simulink model "tqdtqr_rebuild_V3"  (R2021b)
settings: Solver=VariableStepAuto  StartTime=0.0  StopTime=10.0  RelTol=1e-3
undefined symbols (not defined in the file): ATQD_AfterTqMinGain_X_Deg, ATQD_APSCreepBaseTqD_X_kph, ATQD_APSCreepBaseTqD_Y_Deg, ATQD_APSCreepBaseTqR_X_kph, ATQD_APSCreepBaseTqR_Y_Deg, ATQD_APSCreepIterm_X_kph, ATQD_APSCreepIterm_Y_kph, ATQD_APSCreepPterm_X_kph, ATQD_APSCreepPterm_Y_kph, ATQD_APSDecReq_X_kph, ATQD_APSDecReq_Y_mps2, ATQD_APSDecReqCMD_X_kph, ATQD_APSDecReqTs_X_pct, ATQD_APSDecTimeGain_X_Deg, ATQD_APSDecTimeGain_Y_s, ATQD_APSReqLowSpd_X_Deg, ATQD_AutoHoldReleaseBPS_X_Deg, ATQD_AWDLoadTrqnsGain_X_kg, ATQD_AWDLoadTrqnsGain_Y_pct, ATQD_BOSEnBPSPosn_X_kph, ATQD_BOSMap_X_rpm, ATQD_BOSMap_Y_pct, ATQD_CreepBaseTqD_X_kph, ATQD_CreepBaseTqD_Y_Deg, ATQD_CreepBaseTqR_X_kph, ATQD_CreepBaseTqR_Y_Deg, ATQD_CreepBPSDisPosn_X_Deg, ATQD_CreepBPSDisPosnR_X_Deg, ATQD_CreepBPSEnPosn_X_Deg, ATQD_CreepBPSEnPosnR_X_Deg, ATQD_CreepDeltaTq_X_kph, ATQD_CreepIterm_X_kph, ATQD_CreepIterm_Y_kph, ATQD_CreepItermMaxLimit_X_pct, ATQD_CreepPreloadTime_X_kph, ATQD_CreepPreloadTq_X_kph, ATQD_CreepPreloadTq_Y_s, ATQD_CreepProtTq_X_Deg, ATQD_CreepPterm_X_kph, ATQD_CreepPterm_Y_kph, ATQD_CreepRrTqSpRat_X_rpm, ATQD_CreepRrTqSpRat_Y_Nm, ATQD_CreepTargetSpdD_X_pct, ATQD_CreepTargetSpdR_X_pct, ATQD_CreepUpLimitTq_X_rpm, ATQD_DecIneOPDHoldEnDelay_X_Deg, ATQD_DecIneOPDHoldEnDelay_Y_bar, ATQD_ECOTqMapD_X_rpm, ATQD_ECOTqMapD_Y_pct, ATQD_EMTqMapD_X_rpm, ATQD_EMTqMapD_Y_pct, ATQD_EOPDTqMapDCon_X_rpm, ATQD_EOPDTqMapDCon_Y_Deg, ATQD_EstInitVehWeight_X_c, ATQD_FAfterTqCMDGain_X_rpm, ATQD_FAfterTqCMDGain_Y_pct, ATQD_ForceLowSpd_X_Deg, ATQD_ForcePLimitSpd_X_Deg, ATQD_FrLossMAPLowV_X_rpm, ATQD_FrLossMAPLowV_Y_Nm ... (+949)
libraries: simulink x235, hcu_lib x208, tqr x63, tqd x6
(part 23 of 37)

== system tqdtqr_rebuild_V3/Input_Convert/Signal function/SWC1 SWC2 status/SWC2_Subsystem ==
  note: Fail safe switch
  note: Speed Control Mode
  note: Speed Setting Mode
  VINP_SWC2LScrollUpSta_flg : Inport
  VINP_SWC2LScrollDownSta_flg : Inport  Port=2
  VINP_SWC2LScrollPressSta_flg : Inport  Port=3
  VINP_SWC2LADASSta_flg : Inport  Port=4
  VTQD_GearActualPosn_enum : Inport  Port=5
  VVMC_ADASActive_flg : Inport  Port=6
  VVMC_LVDAACCStaInfor_flg : Inport  Port=7
  VVMC_MSAActive_flg : Inport  Port=8
  VINP_ADASACCSta_enum : Inport  Port=9
  VVMC_MeterIndSpeed_raw32 : Inport  Port=10
  VINP_ADASSLIFSpdLim_enum : Inport  Port=11
  task_time_s : Inport  Port=12
  VINP_IVIISAOffsetSpd_enum : Inport  Port=13
  VPMM_PowerSta_enum : Inport  Port=14
  VTQD_ShiftGearPosn_enum : Inport  Port=15
  VVMC_MSACtrlSta_enum : Inport  Port=16
  VINP_Distanceunit_flg : Inport  Port=17
  VINP_IVIACCAdaptiveSta_flg : Inport  Port=18
  VVMC_CCCtrlSta_enum : Inport  Port=19
  VINP_SmartEcoModeSW_flg : Inport  Port=20
  VTQD_LowIdleAccPedal_flg : Inport  Port=21
  Enable : EnablePort
  AND1 : Logic  AllPortsSameDT=off  OutDataTypeStr=boolean
  AND{8,10,12..13,17..18} (6 alike) : Logic  Inputs=3  AllPortsSameDT=off  OutDataTypeStr=boolean
  AND11 : Logic  Inputs=4  AllPortsSameDT=off  OutDataTypeStr=boolean
  AND14 : Logic  Operator=OR  AllPortsSameDT=off  OutDataTypeStr=boolean
  AND16 : Logic  Operator=OR  AllPortsSameDT=off  OutDataTypeStr=boolean
  Add1 : Sum
  Constant1 : Constant  Value=ENUM_ADASACCSTA_OVERRIDE
  Constant{89,92,94..95,110..113} (8 alike) : Constant  Value=FALSE
  Constant116 : Constant  Value=ENUM_GEARACTUALPOSN_D
  Constant117 : Constant  Value=ENUM_SWCBOTTONPRESS_LONGPRESS
  Constant118 : Constant  Value=ENUM_GEARACTUALPOSN_D
  Constant119 : Constant  Value=ENUM_SPDCTRLMODE_MSA
  Constant120 : Constant  Value=ENUM_SWCBOTTONPRESS_SHORTPRESS
  Constant121 : Constant  Value=KTQD_OvrSpdSetDownOffSet_kph
  Constant122 : Constant  Value=ENUM_SWCBOTTONPRESS_LONGPRESS
  Constant123 : Constant  Value=ENUM_SWCBOTTONPRESS_SHORTPRESS
  Constant124 : Constant  Value=ENUM_ADASACCSTA_ACTIVE
  Constant125 : Constant  Value=ENUM_ADASACCSTA_ACTIVE
  Constant126 : Constant  Value=0x0  OutDataTypeStr=uint8
  Constant127 : Constant  Value=ENUM_SPDCTRLMODE_MSA
  Constant128 : Constant  Value=ENUM_SPDCTRLMODE_ACC
  Constant129 : Constant  Value=ENUM_GEARACTUALPOSN_D
  Constant130 : Constant  Value=ENUM_SPDCTRLMODE_MSA
  Constant77 : Constant  Value=KTQD_SpdCtrlMode_enum_ovrdflg
  Constant78 : Constant  Value=KTQD_SpdCtrlMode_enum_ovrdval
  Constant90 : Constant  Value=ENUM_POWERSTA_READY
  Constant91 : Constant  Value=ENUM_SPDCTRLMODE_OFF
  Data Type Conversion : DataTypeConversion  OutDataTypeStr=boolean
  Data Type Conversion4 : DataTypeConversion  OutDataTypeStr=single
  Delay{10..13} (4 alike) : Delay  DelayLength=1  InitialCondition=uint8(0)
      settings: AttributesFormatString=%<InitialCondition>
  Delay5 : Delay  DelayLength=1  InitialCondition=single(0.0)
      settings: AttributesFormatString=%<InitialCondition>
  Detect Decrease2 : simulink/Logic and Bit Operations/Detect Decrease  vinit=boolean(0)  OutDataTypeStr=boolean
  Detect Increase1 : simulink/Logic and Bit Operations/Detect Increase  vinit=boolean(0)  OutDataTypeStr=boolean
  Detect Increase2 : simulink/Logic and Bit Operations/Detect Increase  vinit=boolean(0)  OutDataTypeStr=boolean
  Equal{1,30,41..48,50,52} (12 alike) : RelationalOperator  Operator===  OutDataTypeStr=boolean  RndMeth=Simplest
  Equal{40,49,51,53} (4 alike) : RelationalOperator  Operator=~=  OutDataTypeStr=boolean  RndMeth=Simplest
  L_ScrollPress Behavior : Subsystem
  NOT{1..4} (4 alike) : Logic  Operator=NOT  AllPortsSameDT=off  OutDataTypeStr=boolean
  OR2 : Logic  Operator=OR  Inputs=4  AllPortsSameDT=off  OutDataTypeStr=boolean
  OR{3..8} (6 alike) : Logic  Operator=OR  AllPortsSameDT=off  OutDataTypeStr=boolean
  Relational Operator3 : RelationalOperator  Operator=>  OutDataTypeStr=boolean  RndMeth=Simplest
  Road Speed Limit Convert : Subsystem
  SR_Latch4 : hcu_lib/Basic_Blocks/SR_Latch
  SR_Latch9 : hcu_lib/Basic_Blocks/SR_Latch
  Speed Control Mode : Stateflow chart  TreatAsAtomicUnit=on
  Speed Setting Mode : Subsystem
  Switch{13,15..16,19,23,25..26} (7 alike) : Switch  Criteria=u2 ~= 0
      settings: AttributesFormatString=%<Criteria>
  VTQD_IVIISAOffsetSpdCHOOSE_flg : Subsystem
  VTQD_SWC2ResUpSta_flg : Outport
  VTQD_SWC2SetdownSta_flg : Outport  Port=2
  VTQD_SWC2CancelSta_flg : Outport  Port=3
  VTQD_SWC2LADASSta_flg : Outport  Port=4
  VTQD_SpdLim4SetSpd_raw32 : Outport  Port=5
  VTQD_SpdCtrlMode_enum : Outport  Port=6
  VTQD_SWC2SpdCtrlSta_flg : Outport  Port=7
  VTQD_SWC2SetSpd_kph : Outport  Port=8
  VTQD_SWC2ScrollUpSta_flg : Outport  Port=9
  wires:
  [VVMC_MSACtrlSta_enum] -> L_ScrollPress Behavior/3(VVMC_MSACtrlSta_enum)
  VTQD_LowIdleAccPedal_flg/1 -> [VTQD_LowIdleAccPedal_flg]
  AND1/1 -> AND14/2
  Equal1/1 -> AND14/1
  [VTQD_LowIdleAccPedal_flg] -> NOT3/1
  [VVMC_MSAActive_flg] -> AND1/1
  [VINP_ADASACCSta_enum] -> Equal1/1
  Constant1/1 -> Equal1/2
  NOT3/1 -> AND1/2
  Constant112/1 -> [VDDM_SWC2LScrollPressSta_flg]  "VDDM_SWC2LScrollPressSta_flg"
  Constant110/1 -> [VDDM_SWC2LScrollUpSta_flg]  "VDDM_SWC2LScrollUpSta_flg"
  Constant111/1 -> [VDDM_SWC2LScrollDownSta_flg]  "VDDM_SWC2LScrollDownSta_flg"
  Constant113/1 -> [VDDM_SWC2LADASSta_flg]  "VDDM_SWC2LADASSta_flg"
  VINP_SWC2LScrollDownSta_flg/1 -> [VINP_SWC2LScrollDownSta_flg]
  VTQD_ShiftGearPosn_enum/1 -> [VTQD_ShiftGearPosn_enum]
  VINP_SWC2LScrollPressSta_flg/1 -> [VINP_SWC2LScrollPressSta_flg]
  VINP_IVIISAOffsetSpd_enum/1 -> [VINP_IVIISAOffsetSpd_enum]
  VVMC_ADASActive_flg/1 -> [VVMC_ADASActive_flg]
  VVMC_MSAActive_flg/1 -> [VVMC_MSAActive_flg]
  VVMC_MeterIndSpeed_raw32/1 -> [VVMC_MeterIndSpeed_raw32]
  VVMC_LVDAACCStaInfor_flg/1 -> [VVMC_LVDAACCStaInfor_flg]
  VINP_SWC2LScrollUpSta_flg/1 -> [VINP_SWC2LScrollUpSta_flg]
  VINP_Distanceunit_flg/1 -> [VINP_Distanceunit_flg]
  VVMC_CCCtrlSta_enum/1 -> [VVMC_CCCtrlSta_enum]
  VINP_IVIACCAdaptiveSta_flg/1 -> [VINP_IVIACCAdaptiveSta_flg]
  VINP_SmartEcoModeSW_flg/1 -> [VINP_SmartEcoModeSW_flg]
  VPMM_PowerSta_enum/1 -> [VPMM_PowerSta_enum]
  VINP_SWC2LADASSta_flg/1 -> [VINP_SWC2LADASSta_flg]
  VVMC_MSACtrlSta_enum/1 -> [VVMC_MSACtrlSta_enum]
  task_time_s/1 -> [task_time_s]
  VINP_ADASSLIFSpdLim_enum/1 -> [VINP_ADASSLIFSpdLim_enum]
  VTQD_GearActualPosn_enum/1 -> [VTQD_GearActualPosn_enum]
  VINP_ADASACCSta_enum/1 -> [VINP_ADASACCSta_enum]
  AND16/1 -> AND17/1
  OR2/1 -> [VTQD_SWC2SetDownSta_flg]  "VTQD_SWC2SetdownSta_flg"
  [VTQD_LScrollPressShort_flg] -> Speed Setting Mode/18(VTQD_LScrollPressShort_flg)
  [VTQD_SWC2ScrollUpSta_enum] -> Delay10/1
  [VTQD_GearActualPosn_enum] -> Delay12/1
  Switch25/1 -> [VTQD_SWC2ScrollDownSta_flg]  "VTQD_SWC2ScrollDownSta_flg"
  OR3/1 -> [VTQD_SWC2ResUpSta_flg]  "VTQD_SWC2ResUpSta_flg"
  Switch26/1 -> [VTQD_SWC2LScrollPressSta_flg]  "VTQD_SWC2LScrollPressSta_flg"
  Constant91/1 -> Switch15/3
  [VINP_ADASACCSta_enum] -> Equal50/1
  Constant89/1 -> Switch23/1
  [VDDM_SWC2LScrollDownSta_flg] -> Switch25/2
  [VTQD_ShiftGearPosn_enum] -> Speed Setting Mode/2(VTQD_ShiftGearPosn_enum)
  AND17/1 -> OR2/4, [VTQD_SetRoadSpdLim_flg]  "VTQD_SetRoadSpdLim_flg"
  Constant78/1 -> Switch13/1
  [VTQD_SpdCtrlMode_enum] -> Equal43/1
  [VDDM_SWC2LScrollUpSta_flg] -> Switch23/2
  Constant128/1 -> Equal46/2
  [VTQD_SWC2ScrollUpSta_flg] -> Detect Increase1/1
  OR6/1 -> AND8/3
  Equal51/1 -> OR5/1
  Equal52/1 -> AND12/3
  Constant95/1 -> Switch16/1
  [VINP_SWC2LScrollUpSta_flg] -> Switch23/3
  [VTQD_SWC2ScrollUpSta_enum] -> Equal48/1
  [VTQD_SpdCtrlMode_enum] -> Equal52/1
  AND8/1 -> SR_Latch4/1
  [VTQD_SWC2ScrollUpSta_enum] -> Equal47/1
  Delay10/1 -> Equal41/1
  [VVMC_MSAActive_flg] -> NOT4/1
  SR_Latch9/1 -> OR5/2
  Road Speed Limit Convert/1(VTQD_RoadSpdLim_raw32) -> [VTQD_RoadSpdLim_raw32]
  Equal42/1 -> AND18/2
  [VINP_SWC2LScrollDownSta_flg] -> Switch25/3
  Constant122/1 -> Equal47/2
  Constant119/1 -> Equal44/2
  Equal41/1 -> OR8/1
  [VVMC_MSAActive_flg] -> AND12/2
  [VTQD_SWC2LScrollPressSta_flg] -> L_ScrollPress Behavior/1(VTQD_SWC2LScrollPressSta_flg)
  VTQD_IVIISAOffsetSpdCHOOSE_flg/1(VTQD_IVIISAOffsetSpdCHOOSE_flg) -> [VTQD_IVIISAOffsetSpdCHOOSE_flg]
  [VPMM_PowerSta_enum] -> Equal30/1
  L_ScrollPress Behavior/1(VTQD_LScrollPressShort_flg) -> [VTQD_LScrollPressShort_flg]  "VTQD_LScrollPressShort_flg"
  [VTQD_SpdCtrlMode_enum] -> Equal46/1
  Speed Control Mode/1(VTQD_SpdCtrlMode_enum) -> Switch13/3
  Constant77/1 -> Switch13/2
  [VINP_IVIISAOffsetSpd_enum] -> VTQD_IVIISAOffsetSpdCHOOSE_flg/1(VTQD_IVIISAOffsetSpd_enum)
  Data Type Conversion4/1 -> [VTQD_SWC2SetSpd_kph]  "VTQD_SWC2SetSpd_kph"
  Constant90/1 -> Equal30/2
  Constant94/1 -> Switch26/1
  [VTQD_Set2MeterSpd_flg] -> Speed Setting Mode/16(VTQD_Set2MeterSpd_flg)
  Equal45/1 -> OR8/2
  [VINP_ADASSLIFSpdLim_enum] -> Speed Setting Mode/7(VINP_ADASSLIFSpdLim_enum)
  [VINP_SWC2LScrollPressSta_flg] -> Switch26/3
  Equal44/1 -> AND18/3
  Equal30/1 -> Switch15/2
  [VINP_SWC2LADASSta_flg] -> Switch16/3
  [VDDM_SWC2LScrollPressSta_flg] -> Switch26/2
  AND14/1 -> AND13/2
  AND13/1 -> [VTQD_Set2MeterSpd_flg], OR2/3  "VTQD_Set2MeterSpd_flg"
  [VTQD_GearActualPosn_enum] -> Equal42/1
  Equal40/1 -> AND18/1
  Add1/1 -> Relational Operator3/2
  Constant116/1 -> Equal40/2
  Detect Decrease2/1 -> SR_Latch4/2
  Equal46/1 -> AND10/3
  [VVMC_ADASActive_flg] -> AND8/1
  Delay5/1 -> Add1/2
  [VINP_ADASACCSta_enum] -> Delay13/1
  [VTQD_SWC2CANCELSta_flg] -> NOT1/1
  Constant127/1 -> Equal43/2
  OR8/1 -> Detect Decrease2/1
  [VTQD_SWC2ScrollUpSta_enum] -> Delay11/1
  Constant124/1 -> Equal49/2
  Constant117/1 -> Equal41/2
  L_ScrollPress Behavior/2("VTQD_LScrollPressLong_flg\t") -> [VTQD_LScrollPressLong_flg]  "VTQD_LScrollPressLong_flg"
  [VVMC_MeterIndSpeed_raw32] -> Relational Operator3/1
  Constant123/1 -> Equal48/2
  Constant125/1 -> Equal50/2
  Constant120/1 -> Equal45/2
  [VTQD_LScrollPressLong_flg] -> AND11/2
  [VTQD_SWC2SetSpd_kph] -> Delay5/1
  Equal53/1 -> AND17/3
  Constant126/1 -> Equal53/2
  Equal47/1 -> OR4/1
  OR5/1 -> [VTQD_SWC2CANCELSta_flg]  "VTQD_SWC2CancelSta_flg"
  [VVMC_MSAActive_flg] -> AND16/2
  [VTQD_GearActualPosn_enum] -> Equal51/1
  AND12/1 -> SR_Latch9/1
  Constant92/1 -> Switch25/1
  Speed Setting Mode/2(VTQD_SWC2ScrollUpSta_enum) -> [VTQD_SWC2ScrollUpSta_enum]
  Equal49/1 -> AND10/1
  [VVMC_ADASActive_flg] -> AND16/1
  [VTQD_LScrollPressLong_flg] -> AND12/1
  Constant121/1 -> Add1/1
  [VPMM_PowerSta_enum] -> Speed Control Mode/1(VPMM_PowerSta_enum)
  Constant129/1 -> Equal51/2
  [VTQD_SpdLim4SetSpd_raw32] -> Speed Setting Mode/12(VTQD_SpdLim4SetSpd_raw32)
  NOT1/1 -> AND11/1
  AND10/1 -> OR2/2
  [VINP_ADASSLIFSpdLim_enum] -> Road Speed Limit Convert/1(VINP_ADASSLIFSpdLim_enum)
  [VTQD_SWC2LADASSta_flg] -> Speed Control Mode/4(VTQD_SWC2LADASSta_flg)
  [VINP_Distanceunit_flg] -> Road Speed Limit Convert/4(VINP_Distanceunit_flg)
  Delay12/1 -> Equal40/1
  NOT4/1 -> AND11/4
  [VTQD_ShiftGearPosn_enum] -> Road Speed Limit Convert/5(VTQD_ShiftGearPosn_enum)
  [VVMC_MSACtrlSta_enum] -> Speed Control Mode/5(VVMC_MSACtrlSta_enum)
  Relational Operator3/1 -> AND13/1
  [VTQD_ShiftGearPosn_enum] -> Speed Control Mode/3(VTQD_ShiftGearPosn_enum)
  [VVMC_CCCtrlSta_enum] -> Speed Setting Mode/5(VVMC_CCCtrlSta_enum)
  Equal50/1 -> AND10/2
  [VTQD_SetRoadSpdLim_flg] -> OR7/2
  [VTQD_SpdCtrlMode_enum] -> Equal44/1
  [VVMC_MSACtrlSta_enum] -> Speed Setting Mode/6(VVMC_MSACtrlSta_enum)
  [VTQD_SpdCtrlMode_enum] -> Speed Setting Mode/3(VTQD_SpdCtrlMode_enum)
  [VTQD_SetRoadSpdLim_flg] -> Speed Setting Mode/17(VTQD_SetRoadSpdLim_flg)
  Equal43/1 -> AND11/3
  [task_time_s] -> L_ScrollPress Behavior/2(TASK_TIME)
  Detect Increase1/1 -> OR6/1
  OR7/1 -> Switch19/2
  OR4/1 -> AND13/3
  [VTQD_SWC2ScrollUpSta_flg] -> Speed Setting Mode/8(VTQD_SWC2ScrollUpSta_flg)
  [task_time_s] -> Speed Setting Mode/10(task_time_s)
  Switch15/1 -> [VTQD_SpdCtrlMode_enum]  "VTQD_SpdCtrlMode_enum"
  [VTQD_SWC2ScrollDownSta_flg] -> Speed Setting Mode/9(VTQD_SWC2ScrollDownSta_flg)
  [VVMC_LVDAACCStaInfor_flg] -> Speed Setting Mode/11(VVMC_LVDAACCStatusInformation_flg)
  [VINP_IVIACCAdaptiveSta_flg] -> OR7/1
  [VINP_Distanceunit_flg] -> Speed Setting Mode/13(VINP_Distanceunit_flg)
  [VINP_SmartEcoModeSW_flg] -> Speed Setting Mode/14(VINP_SmartEcoModeSW_flg)
  [VINP_IVIACCAdaptiveSta_flg] -> Speed Setting Mode/15(VINP_IVIACCAdaptiveSta_flg)
  [VINP_ADASACCSta_enum] -> Speed Setting Mode/4(VINP_ADASACCSta_enum)
  [VTQD_RoadSpdLim_raw32] -> Switch19/1
  [VTQD_LScrollPressLong_flg] -> Speed Control Mode/2(VTQD_LScrollPressLong_flg)
  Delay13/1 -> Equal49/1
  [VVMC_LVDAACCStaInfor_flg] -> AND8/2
  AND18/1 -> OR3/1
  [VTQD_IVIISAOffsetSpdCHOOSE_flg] -> Road Speed Limit Convert/3(VTQD_IVIISAOffsetSpdCHOOSE_flg)
  [VTQD_SWC2LScrollPressSta_flg] -> NOT2/1
  [VVMC_MeterIndSpeed_raw32] -> Switch19/3
  Equal48/1 -> OR4/2
  Constant118/1 -> Equal42/2
  [VTQD_LScrollPressShort_flg] -> AND17/2
  Switch16/1 -> [VTQD_SWC2LADASSta_flg]  "VTQD_SWC2LADASSta_flg"
  NOT2/1 -> SR_Latch9/2
  [VVMC_MeterIndSpeed_raw32] -> Speed Setting Mode/19(VVMC_MeterIndSpeed_raw32)
  [VTQD_SWC2LADASSta_flg] -> Detect Increase2/1
  SR_Latch4/1 -> OR3/2
  [VINP_ADASSLIFSpdLim_enum] -> Equal53/1
  Delay11/1 -> Equal45/1
  AND11/1 -> OR2/1
  [VDDM_SWC2LADASSta_flg] -> Switch16/2
  Switch13/1 -> Switch15/1
  [VPMM_PowerSta_enum] -> Speed Setting Mode/1(VPMM_PowerSta_enum)
  [VINP_IVIISAOffsetSpd_enum] -> Road Speed Limit Convert/2(VINP_IVIISAOffsetSpd_enum)
  Switch23/1 -> [VTQD_SWC2ScrollUpSta_flg]  "VTQD_SWC2ScrollUpSta_flg"
  Switch19/1 -> [VTQD_SpdLim4SetSpd_raw32]  "VTQD_SpdLim4SetSpd_raw32"
  Constant130/1 -> Equal52/2
  Detect Increase2/1 -> OR6/2
  [VTQD_SWC2ResUpSta_flg] -> VTQD_SWC2ResUpSta_flg/1
  [VTQD_SpdCtrlMode_enum] -> VTQD_SpdCtrlMode_enum/1
  [VTQD_SWC2SetSpd_kph] -> VTQD_SWC2SetSpd_kph/1
  [VTQD_SWC2SpdCtrlSta_flg] -> VTQD_SWC2SpdCtrlSta_flg/1
  [VTQD_SpdLim4SetSpd_raw32] -> VTQD_SpdLim4SetSpd_raw32/1
  [VTQD_SWC2SetDownSta_flg] -> VTQD_SWC2SetdownSta_flg/1
  [VTQD_SWC2CANCELSta_flg] -> VTQD_SWC2CancelSta_flg/1
  [VTQD_SWC2ScrollUpSta_flg] -> VTQD_SWC2ScrollUpSta_flg/1
  [VTQD_SWC2LADASSta_flg] -> VTQD_SWC2LADASSta_flg/1
  Speed Control Mode/2(VTQD_SpdCtrlSta_flg) -> Data Type Conversion/1
  Data Type Conversion/1 -> [VTQD_SWC2SpdCtrlSta_flg]  "VTQD_SWC2SpdCtrlSta_flg"
  Speed Setting Mode/1(VTQD_SetSpd_kph) -> Data Type Conversion4/1

== system tqdtqr_rebuild_V3/Input_Convert/Signal function/SWC1 SWC2 status/SWC_Subsystem ==
  note: Speed Setting Mode
  note: Speed Control Mode
  VDDM_SWCResUpSta_flg : Inport
  VINP_SWCResUpSta_flg : Inport  Port=2
  VDDM_SWCSetdownSta_flg : Inport  Port=3
  VINP_SWCSetdownSta_flg : Inport  Port=4
  VDDM_SWCACCSta_flg : Inport  Port=5
  VINP_SWCACCSta_flg : Inport  Port=6
  VDDM_SWCCANCELSta_flg : Inport  Port=7
  VINP_SWCCANCELSta_flg : Inport  Port=8
  VTQD_IVIISAOffsetSpd_enum : Inport  Port=9
  VPMM_PowerSta_enum : Inport  Port=10
  VINP_ADASACCSta_enum : Inport  Port=11
  VINP_ADASISASta_enum : Inport  Port=12
  VTQD_ShiftGearPosn_enum : Inport  Port=13
  VVMC_CCCtrlSta_enum : Inport  Port=14
  VVMC_MSACtrlSta_enum : Inport  Port=15
  VINP_ADASVehSpdLim_kph : Inport  Port=16
  task_time_s : Inport  Port=17
  VVMC_LVDAACCStatusInformation_flg : Inport  Port=18
  VVMC_ACCObjDist_m : Inport  Port=19
  VVMC_MeterIndSpeed_raw32 : Inport  Port=20
  VINP_Distanceunit_flg : Inport  Port=21
  VINP_SmartEcoModeSW_flg : Inport  Port=22
  VVMC_SetACCDisableAPS_flg : Inport  Port=23
  Enable : EnablePort
  Constant77 : Constant  Value=KTQD_SpdCtrlMode_enum_ovrdflg
  Constant78 : Constant  Value=KTQD_SpdCtrlMode_enum_ovrdval
  Constant{89,92,94..95} (4 alike) : Constant  Value=FALSE
  Constant90 : Constant  Value=ENUM_POWERSTA_READY
  Constant91 : Constant  Value=ENUM_SPDCTRLMODE_OFF
  Data Type Conversion : DataTypeConversion  OutDataTypeStr=boolean
  Data Type Conversion4 : DataTypeConversion  OutDataTypeStr=single
  Equal30 : RelationalOperator  Operator===  OutDataTypeStr=boolean  RndMeth=Simplest
  SpdCtrlBotton Behavior : Subsystem
  Speed Control Mode : Stateflow chart  TreatAsAtomicUnit=on
  Speed Setting Mode : Subsystem
  Switch{13,15..16,23,25..26} (6 alike) : Switch  Criteria=u2 ~= 0
      settings: AttributesFormatString=%<Criteria>
  VTQD_IVIISAOffsetSpdCHOOSE_flg : Subsystem
  VTQD_SWCResUpSta_flg : Outport
  VTQD_SWCSetdownSta_flg : Outport  Port=2
  VTQD_SWCCancelSta_flg : Outport  Port=3
  VTQD_SWCSpdCtrlMode_enum : Outport  Port=4
  VTQD_SWCSpdCtrlSta_flg : Outport  Port=5
  VTQD_SWC1SetSpd_kph : Outport  Port=6
  wires:
  [VINP_ADASACCSta_enum] -> Speed Setting Mode/4(VINP_ADASACCSta_enum)
  [VINP_ADASACCSta_enum] -> Speed Control Mode/4(VINP_ADASACCSta_enum)
  VINP_ADASACCSta_enum/1 -> [VINP_ADASACCSta_enum]
  [VPMM_PowerSta_enum] -> Speed Setting Mode/1(VPMM_PowerSta_enum)
  [VPMM_PowerSta_enum] -> Speed Control Mode/1(VPMM_PowerSta_enum)
  VPMM_PowerSta_enum/1 -> [VPMM_PowerSta_enum]
  [VTQD_ShiftGearPosn_enum] -> Speed Setting Mode/2(VTQD_ShiftGearPosn_enum)
  [VTQD_ShiftGearPosn_enum] -> Speed Control Mode/7(VTQD_ShiftGearPosn_enum)
  VTQD_ShiftGearPosn_enum/1 -> [VTQD_ShiftGearPosn_enum]
  [task_time_s] -> Speed Setting Mode/10(task_time_s)
  task_time_s/1 -> [task_time_s]
  Switch15/1 -> [VTQD_SpdCtrlMode_enum]  "VTQD_SWCSpdCtrlMode_enum"
  Constant90/1 -> Equal30/2
  Equal30/1 -> Switch15/2
  [VTQD_IVIISAOffsetSpdCHOOSE_flg] -> Speed Control Mode/6(VTQD_IVIISAOffsetSpdCHOOSE_flg)
  Switch25/1 -> [VTQD_SWCSetdownSta_flg]  "VTQD_SWCSetdownSta_flg"
  Switch23/1 -> [VTQD_SWCResUpSta_flg]  "VTQD_SWCResUpSta_flg"
  [VPMM_PowerSta_enum] -> Equal30/1
  Speed Control Mode/1(VTQD_SpdCtrlMode_enum) -> Switch13/3
  VTQD_IVIISAOffsetSpdCHOOSE_flg/1(VTQD_IVIISAOffsetSpdCHOOSE_flg) -> [VTQD_IVIISAOffsetSpdCHOOSE_flg]
  Constant94/1 -> Switch26/1
  Constant78/1 -> Switch13/1
  SpdCtrlBotton Behavior/1(VTQD_SpdCtrlShortP_flg) -> [VTQD_SpdCtrlShortP_flg]  "VTQD_SpdCtrlShortP_flg"
  [VTQD_SWCACCSta_flg] -> SpdCtrlBotton Behavior/1(SWC_ACC_Sta)
  [VTQD_SWCSetdownSta_flg] -> Speed Setting Mode/9(VTQD_SWCSetDownSta_flg)
  [VTQD_SpdCtrlShortP_flg] -> Speed Control Mode/2(VTQD_SpdCtrlShortP_flg)
  Switch16/1 -> [VTQD_SWCCancelSta_flg]  "VTQD_SWCCancelSta_flg"
  Switch13/1 -> Switch15/1
  [VTQD_SpdCtrlLongP_flg] -> Speed Control Mode/3(VTQD_SpdCtrlLongP_flg)
  Constant95/1 -> Switch16/1
  Constant91/1 -> Switch15/3
  Switch26/1 -> [VTQD_SWCACCSta_flg]  "VTQD_SWCACCSta_flg"
  [VTQD_SWCResUpSta_flg] -> Speed Setting Mode/8(VTQD_SWCResUpSta_flg)
  Constant92/1 -> Switch25/1
  SpdCtrlBotton Behavior/2("VTQD_SpdCtrlLongP_flg\t") -> [VTQD_SpdCtrlLongP_flg]  "VTQD_SpdCtrlLongP_flg"
  [task_time_s] -> SpdCtrlBotton Behavior/2(TASK_TIME)
  Constant89/1 -> Switch23/1
  Speed Setting Mode/1(VTQD_SetSpd_kph) -> Data Type Conversion4/1
  Constant77/1 -> Switch13/2
  [VTQD_SpdCtrlMode_enum] -> Speed Setting Mode/3(VTQD_SpdCtrlMode_enum)
  VDDM_SWCACCSta_flg/1 -> [VDDM_SWCACCSta_flg]
  [VDDM_SWCACCSta_flg] -> Switch26/2
  VINP_SWCACCSta_flg/1 -> [VINP_SWCACCSta_flg]
  [VINP_SWCACCSta_flg] -> Switch26/3
  [VTQD_IVIISAOffsetSpd_enum] -> VTQD_IVIISAOffsetSpdCHOOSE_flg/1(VTQD_IVIISAOffsetSpd_enum)
  VTQD_IVIISAOffsetSpd_enum/1 -> [VTQD_IVIISAOffsetSpd_enum]
  VINP_ADASISASta_enum/1 -> [VINP_ADASISASta_enum]
  [VINP_ADASISASta_enum] -> Speed Control Mode/5(VINP_ADASISASta_enum)
  [VTQD_SpdCtrlMode_enum] -> VTQD_SWCSpdCtrlMode_enum/1
  Data Type Conversion4/1 -> [VTQD_SWC1SetSpd_kph]  "VTQD_SWC1SetSpd_kph"
  [VTQD_SWC1SetSpd_kph] -> VTQD_SWC1SetSpd_kph/1
  [VTQD_SWCCancelSta_flg] -> VTQD_SWCCancelSta_flg/1
  [VTQD_SWCSetdownSta_flg] -> VTQD_SWCSetdownSta_flg/1
  [VTQD_SWCResUpSta_flg] -> VTQD_SWCResUpSta_flg/1
  VDDM_SWCResUpSta_flg/1 -> [VDDM_SWCResUpSta_flg]
  [VDDM_SWCResUpSta_flg] -> Switch23/2
  VINP_SWCResUpSta_flg/1 -> [VINP_SWCResUpSta_flg]
  [VINP_SWCResUpSta_flg] -> Switch23/3
  VDDM_SWCSetdownSta_flg/1 -> [VDDM_SWCSetdownSta_flg]
  [VDDM_SWCSetdownSta_flg] -> Switch25/2
  VINP_SWCSetdownSta_flg/1 -> [VINP_SWCSetdownSta_flg]
  [VINP_SWCSetdownSta_flg] -> Switch25/3
  VDDM_SWCCANCELSta_flg/1 -> [VDDM_SWCCANCELSta_flg]
  [VDDM_SWCCANCELSta_flg] -> Switch16/2
  VINP_SWCCANCELSta_flg/1 -> [VINP_SWCCANCELSta_flg]
  [VINP_SWCCANCELSta_flg] -> Switch16/3
  VVMC_CCCtrlSta_enum/1 -> [VVMC_CCCtrlSta_enum]
  [VVMC_CCCtrlSta_enum] -> Speed Setting Mode/5(VVMC_CCCtrlSta_enum)
  VVMC_MSACtrlSta_enum/1 -> [VVMC_MSACtrlSta_enum]
  [VVMC_MSACtrlSta_enum] -> Speed Setting Mode/6(VVMC_MSACtrlSta_enum)
  VINP_ADASVehSpdLim_kph/1 -> [VINP_ADASVehSpdLim_kph]
  [VINP_ADASVehSpdLim_kph] -> Speed Setting Mode/7(VINP_ADASVehSpdLim_kph)
  [VVMC_LVDAACCStatusInformation_flg] -> Speed Setting Mode/11(VVMC_LVDAACCStatusInformation_flg)
  VVMC_LVDAACCStatusInformation_flg/1 -> [VVMC_LVDAACCStatusInformation_flg]
  VVMC_ACCObjDist_m/1 -> [VVMC_ACCObjDist_m]
  [VVMC_ACCObjDist_m] -> Speed Setting Mode/12(VVMC_ACCObjDist_m)
  VVMC_MeterIndSpeed_raw32/1 -> [VVMC_MeterIndSpeed_raw32]
  [VVMC_MeterIndSpeed_raw32] -> Speed Setting Mode/13(VVMC_MeterIndSpeed_raw32)
  [VINP_Distanceunit_flg] -> Speed Setting Mode/14(VINP_Distanceunit_flg)
  VINP_Distanceunit_flg/1 -> [VINP_Distanceunit_flg]
  VINP_SmartEcoModeSW_flg/1 -> [VINP_SmartEcoModeSW_flg]
  [VINP_SmartEcoModeSW_flg] -> Speed Setting Mode/15(VINP_SmartEcoModeSW_flg)
  VVMC_SetACCDisableAPS_flg/1 -> [VVMC_SetACCDisableAPS_flg]
  [VVMC_SetACCDisableAPS_flg] -> Speed Setting Mode/16(VVMC_SetACCDisableAPS_flg)
  [VTQD_SWCSpdCtrlSta_flg] -> VTQD_SWCSpdCtrlSta_flg/1
  Speed Control Mode/2(VTQD_SpdCtrlSta_flg) -> Data Type Conversion/1
  Data Type Conversion/1 -> [VTQD_SWCSpdCtrlSta_flg]  "VTQD_SWCSpdCtrlSta_flg"

== system tqdtqr_rebuild_V3/Input_Convert/Signal function/ShiftModule/Determin Gear State Configuration ==
  note: R to N
  note: N to R
  note: R to D
  note: D to R
  note: D to N
  note: N to D
  note: R to P
  note: P to R
  note: D to P
  note: P to D
  note: N to P
  note: P to N
  VTQD_BrkSwSta_flg : Inport
  VTQD_GearShiftCMD_enum : Inport  Port=2
  VINP_VehSpeed_kph : Inport  Port=3
  VTQD_PwrStaAllowDR_flg : Inport  Port=4
  VTQD_PwrStaAllowPN_flg : Inport  Port=5
  VTQD_TMRotateDirction_enum : Inport  Port=6
  VTQD_EPBCarWashMode_flg : Inport  Port=7
  VVMC_APSActive_flg : Inport  Port=8
  VTQD_ForceP_flg : Inport  Port=9
  VTQD_IVIRockModeEn_flg : Inport  Port=10
  VTQD_MaxShaftSpd_rpm : Inport  Port=11
  VTQD_ExitP_flg : Inport  Port=12
  VTQD_EnterP_flg : Inport  Port=13
  Constant : Constant  Value=ENUM_GEARSHIFTCMD_N
  Constant1 : Constant  Value=ENUM_GEARSHIFTCMD_P
  Constant10 : Constant  Value=ENUM_TMROTATEDIRECTACT_REVERSE
  Constant11 : Constant  Value=ENUM_GEARSHIFTCMD_N
  Constant12 : Constant  Value=ENUM_GEARSHIFTCMD_R
  Constant13 : Constant  Value=KTQD_VehSpdRev_kph
  Constant14 : Constant  Value=KTQD_RockVehSpdRev_rpm
  Constant15 : Constant  Value=ENUM_GEARSHIFTCMD_D
  Constant16 : Constant  Value=KTQD_VehSpdRev_kph
  Constant17 : Constant  Value=KTQD_RockVehSpdRev_rpm
  Constant18 : Constant  Value=ENUM_GEARSHIFTCMD_R
  Constant19 : Constant  Value=ENUM_TMROTATEDIRECTACT_FORWARD
  Constant2 : Constant  Value=KTQD_VehSpd2P_kph
  Constant20 : Constant  Value=ENUM_GEARSHIFTCMD_N
  Constant3 : Constant  Value=ENUM_GEARSHIFTCMD_D
  Constant4 : Constant  Value=ENUM_GEARSHIFTCMD_P
  Constant5 : Constant  Value=KTQD_VehSpd2P_kph
  Constant6 : Constant  Value=ENUM_GEARSHIFTCMD_R
  Constant7 : Constant  Value=KTQD_VehSpd2P_kph
  Constant8 : Constant  Value=ENUM_GEARSHIFTCMD_P
  Constant9 : Constant  Value=ENUM_GEARSHIFTCMD_D
  Delay4 : Delay  DelayLength=1  InitialCondition=boolean(0)
      settings: AttributesFormatString=%<InitialCondition>
  Delay5 : Delay  DelayLength=1  InitialCondition=boolean(0)
      settings: AttributesFormatString=%<InitialCondition>
  Equal{,1,3..4,6..7,9,11,14,17,19..20} (12 alike) : RelationalOperator  Operator===  OutDataTypeStr=boolean  RndMeth=Simplest
  Equal10 : RelationalOperator  Operator=~=  OutDataTypeStr=boolean  RndMeth=Simplest
  Equal{2,5,8,12..13,15..16} (7 alike) : RelationalOperator  Operator=<=  OutDataTypeStr=boolean  RndMeth=Simplest
  Equal18 : RelationalOperator  Operator=~=  OutDataTypeStr=boolean  RndMeth=Simplest
  Logical Operator{,5..6,10,12,15,23,26} (8 alike) : Logic  Operator=OR  AllPortsSameDT=off  OutDataTypeStr=boolean
  Logical Operator{1,7,11,16,18,29,31} (7 alike) : Logic  Operator=NOT  AllPortsSameDT=off  OutDataTypeStr=boolean
  Logical Operator13 : Logic  Inputs=5  AllPortsSameDT=off  OutDataTypeStr=boolean
  Logical Operator14 : Logic  Inputs=3  AllPortsSameDT=off  OutDataTypeStr=boolean
  Logical Operator{2,4,17,21,27} (5 alike) : Logic  Inputs=4  AllPortsSameDT=off  OutDataTypeStr=boolean
  Logical Operator{19..20,24,28,32} (5 alike) : Logic  Operator=OR  Inputs=3  AllPortsSameDT=off  OutDataTypeStr=boolean
  Logical Operator22 : Logic  AllPortsSameDT=off  OutDataTypeStr=boolean
  Logical Operator25 : Logic  AllPortsSameDT=off  OutDataTypeStr=boolean
  Logical Operator3 : Logic  AllPortsSameDT=off  OutDataTypeStr=boolean
  Logical Operator30 : Logic  Inputs=5  AllPortsSameDT=off  OutDataTypeStr=boolean
  Logical Operator8 : Logic  Inputs=5  AllPortsSameDT=off  OutDataTypeStr=boolean
  Logical Operator9 : Logic  Inputs=3  AllPortsSameDT=off  OutDataTypeStr=boolean
  VTQD_GearP2N_flg : Outport
  VTQD_GearN2P_flg : Outport  Port=2
  VTQD_GearP2D_flg : Outport  Port=3
  VTQD_GearD2P_flg : Outport  Port=4
  VTQD_GearP2R_flg : Outport  Port=5
  VTQD_GearR2P_flg : Outport  Port=6
  VTQD_GearN2D_flg : Outport  Port=7
  VTQD_GearD2N_flg : Outport  Port=8
  VTQD_GearD2R_flg : Outport  Port=9
  VTQD_GearR2D_flg : Outport  Port=10
  VTQD_GearN2R_flg : Outport  Port=11
  VTQD_GearR2N_flg : Outport  Port=12
  wires:
  VTQD_BrkSwSta_flg/1 -> [VTQD_BrkSwSta_flg]
  VTQD_GearShiftCMD_enum/1 -> [VTQD_GearShiftCMD_enum]
  VINP_VehSpeed_kph/1 -> [VINP_VehSpeed_kph]
  VTQD_PwrStaAllowDR_flg/1 -> [VTQD_PwrStaAllowDR_flg]
  VTQD_PwrStaAllowPN_flg/1 -> [VTQD_PwrStaAllowPN_flg]
  VTQD_TMRotateDirction_enum/1 -> [VTQD_TMRotateDirction_enum]
  VTQD_EPBCarWashMode_flg/1 -> [VTQD_EPBCarWashMode_flg]
  VVMC_APSActive_flg/1 -> [VVMC_APSActive_flg]
  VTQD_ForceP_flg/1 -> [VTQD_ForceP_flg]
  VTQD_IVIRockModeEn_flg/1 -> [VTQD_IVIRockModeEn_flg]
  VTQD_MaxShaftSpd_rpm/1 -> [VTQD_MaxShaftSpd_rpm]
  [VTQD_GearShiftCMD_enum] -> Equal/1
  Constant/1 -> Equal/2
  [VTQD_BrkSwSta_flg] -> Logical Operator/1
  [VVMC_APSActive_flg] -> Logical Operator/2
  [VTQD_ForceP_flg] -> Logical Operator1/1
  Equal/1 -> Logical Operator2/1
  [VTQD_PwrStaAllowPN_flg] -> Logical Operator2/2
  Logical Operator/1 -> Logical Operator2/3
  Logical Operator2/1 -> Logical Operator3/1
  Logical Operator1/1 -> Logical Operator3/2
  Logical Operator3/1 -> [VTQD_GearP2N_flg]  "VTQD_GearP2N_flg"
  [VTQD_GearP2N_flg] -> VTQD_GearP2N_flg/1
  [VTQD_GearShiftCMD_enum] -> Equal1/1
  Constant1/1 -> Equal1/2
  [VINP_VehSpeed_kph] -> Equal2/1
  Constant2/1 -> Equal2/2
  Equal1/1 -> Logical Operator4/1
  [VTQD_PwrStaAllowPN_flg] -> Logical Operator4/2
  Equal2/1 -> Logical Operator4/3
  [VTQD_ForceP_flg] -> Logical Operator5/2
  Logical Operator4/1 -> Logical Operator5/1
  Logical Operator5/1 -> [VTQD_GearN2P_flg]  "VTQD_GearN2P_flg"
  [VTQD_GearN2P_flg] -> VTQD_GearN2P_flg/1
  [VTQD_GearShiftCMD_enum] -> Equal3/1
  Constant3/1 -> Equal3/2
  [VTQD_BrkSwSta_flg] -> Logical Operator6/1
  [VVMC_APSActive_flg] -> Logical Operator6/2
  [VTQD_ForceP_flg] -> Logical Operator7/1
  Equal3/1 -> Logical Operator8/1
  [VTQD_PwrStaAllowDR_flg] -> Logical Operator8/2
  Logical Operator6/1 -> Logical Operator8/3
  Logical Operator7/1 -> Logical Operator8/5
  Logical Operator8/1 -> [VTQD_GearP2D_flg]  "VTQD_GearP2D_flg"
  [VTQD_GearP2D_flg] -> VTQD_GearP2D_flg/1
  [VTQD_GearShiftCMD_enum] -> Equal4/1
  Constant4/1 -> Equal4/2
  Constant5/1 -> Equal5/2
  Equal4/1 -> Logical Operator9/1
  [VTQD_PwrStaAllowPN_flg] -> Logical Operator9/2
  Equal5/1 -> Logical Operator9/3
  Logical Operator9/1 -> Logical Operator10/1
  [VTQD_ForceP_flg] -> Logical Operator10/2
  Logical Operator10/1 -> [VTQD_GearD2P_flg]  "VTQD_GearD2P_flg"
  [VTQD_GearD2P_flg] -> VTQD_GearD2P_flg/1
  [VTQD_GearShiftCMD_enum] -> Equal6/1
  Constant6/1 -> Equal6/2
  [VTQD_ForceP_flg] -> Logical Operator11/1
  [VTQD_BrkSwSta_flg] -> Logical Operator12/1
  [VVMC_APSActive_flg] -> Logical Operator12/2
  Equal6/1 -> Logical Operator13/1
  [VTQD_PwrStaAllowDR_flg] -> Logical Operator13/2
  Logical Operator12/1 -> Logical Operator13/3
  Logical Operator11/1 -> Logical Operator13/5
  Logical Operator13/1 -> [VTQD_GearP2R_flg]  "VTQD_GearP2R_flg"
  [VTQD_GearP2R_flg] -> VTQD_GearP2R_flg/1
  [VINP_VehSpeed_kph] -> Equal5/1
  [VTQD_GearShiftCMD_enum] -> Equal7/1
  Constant8/1 -> Equal7/2
  [VINP_VehSpeed_kph] -> Equal8/1
  Constant7/1 -> Equal8/2
  Equal7/1 -> Logical Operator14/1
  [VTQD_PwrStaAllowPN_flg] -> Logical Operator14/2
  Equal8/1 -> Logical Operator14/3
  Logical Operator14/1 -> Logical Operator15/1
  [VTQD_ForceP_flg] -> Logical Operator15/2
  Logical Operator15/1 -> [VTQD_GearR2P_flg]  "VTQD_GearR2P_flg"
  [VTQD_GearR2P_flg] -> VTQD_GearR2P_flg/1
  [VTQD_GearShiftCMD_enum] -> Equal9/1
  Constant9/1 -> Equal9/2
  [VTQD_TMRotateDirction_enum] -> Equal10/1
  Constant10/1 -> Equal10/2
  [VTQD_EPBCarWashMode_flg] -> Logical Operator16/1
  Equal9/1 -> Logical Operator17/1
  [VTQD_PwrStaAllowDR_flg] -> Logical Operator17/2
  Equal10/1 -> Logical Operator17/3
  Logical Operator16/1 -> Logical Operator17/4
  Logical Operator17/1 -> [VTQD_GearN2D_flg]  "VTQD_GearN2D_flg"
  [VTQD_GearN2D_flg] -> VTQD_GearN2D_flg/1
  [VTQD_PwrStaAllowDR_flg] -> Logical Operator18/1
  Logical Operator18/1 -> Logical Operator19/2
  [VTQD_EPBCarWashMode_flg] -> Logical Operator19/3
  Logical Operator19/1 -> [VTQD_GearD2N_flg]  "VTQD_GearD2N_flg"
  [VTQD_GearD2N_flg] -> VTQD_GearD2N_flg/1
  Constant12/1 -> Equal11/2
  [VTQD_GearShiftCMD_enum] -> Equal11/1
  [VTQD_BrkSwSta_flg] -> Logical Operator20/1
  [VVMC_APSActive_flg] -> Logical Operator20/2
  [VTQD_IVIRockModeEn_flg] -> Logical Operator20/3
  [VINP_VehSpeed_kph] -> Equal12/1
  Constant13/1 -> Equal12/2
  [VTQD_MaxShaftSpd_rpm] -> Equal13/1
  Constant14/1 -> Equal13/2
  Equal11/1 -> Logical Operator21/1
  Logical Operator20/1 -> Logical Operator21/3
  [VTQD_PwrStaAllowDR_flg] -> Logical Operator21/2
  Equal13/1 -> Logical Operator22/2
  [VTQD_IVIRockModeEn_flg] -> Logical Operator22/1
  Equal12/1 -> Logical Operator23/1
  Logical Operator22/1 -> Logical Operator23/2
  Logical Operator23/1 -> Logical Operator21/4
  Logical Operator21/1 -> [VTQD_GearD2R_flg]  "VTQD_GearD2R_flg"
  [VTQD_GearD2R_flg] -> VTQD_GearD2R_flg/1
  [VTQD_GearShiftCMD_enum] -> Equal14/1
  Constant15/1 -> Equal14/2
  [VTQD_BrkSwSta_flg] -> Logical Operator24/1
  [VTQD_IVIRockModeEn_flg] -> Logical Operator24/3
  [VVMC_APSActive_flg] -> Logical Operator24/2
  Constant16/1 -> Equal15/2
  [VINP_VehSpeed_kph] -> Equal15/1
  Equal15/1 -> Logical Operator26/1
  Constant17/1 -> Equal16/2
  Equal16/1 -> Logical Operator25/2
  [VTQD_MaxShaftSpd_rpm] -> Equal16/1
  [VTQD_IVIRockModeEn_flg] -> Logical Operator25/1
  Logical Operator25/1 -> Logical Operator26/2
  Logical Operator26/1 -> Logical Operator27/4
  Logical Operator24/1 -> Logical Operator27/3
  [VTQD_PwrStaAllowDR_flg] -> Logical Operator27/2
  Equal14/1 -> Logical Operator27/1
  Logical Operator27/1 -> [VTQD_GearR2D_flg]  "VTQD_GearR2D_flg"
  [VTQD_GearR2D_flg] -> VTQD_GearR2D_flg/1
  [VTQD_GearShiftCMD_enum] -> Equal17/1
  Constant18/1 -> Equal17/2
  [VTQD_TMRotateDirction_enum] -> Equal18/1
  Constant19/1 -> Equal18/2
  Logical Operator28/1 -> Logical Operator30/4
  [VVMC_APSActive_flg] -> Logical Operator28/2
  [VTQD_IVIRockModeEn_flg] -> Logical Operator28/3
  [VTQD_BrkSwSta_flg] -> Logical Operator28/1
  [VTQD_EPBCarWashMode_flg] -> Logical Operator29/1
  Equal17/1 -> Logical Operator30/1
  [VTQD_PwrStaAllowDR_flg] -> Logical Operator30/2
  Equal18/1 -> Logical Operator30/3
  Logical Operator29/1 -> Logical Operator30/5
  Logical Operator30/1 -> [VTQD_GearN2R_flg]  "VTQD_GearN2R_flg"
  [VTQD_GearN2R_flg] -> VTQD_GearN2R_flg/1
  [VTQD_GearShiftCMD_enum] -> Equal19/1
  Constant20/1 -> Equal19/2
  [VTQD_PwrStaAllowDR_flg] -> Logical Operator31/1
  Equal19/1 -> Logical Operator32/1
  Logical Operator31/1 -> Logical Operator32/2
  [VTQD_EPBCarWashMode_flg] -> Logical Operator32/3
  Logical Operator32/1 -> [VTQD_GearR2N_flg]  "VTQD_GearR2N_flg"
  [VTQD_GearR2N_flg] -> VTQD_GearR2N_flg/1
  VTQD_ExitP_flg/1 -> Delay4/1
  Delay4/1 -> [VTQD_ExitP_flg]
  VTQD_EnterP_flg/1 -> Delay5/1
  Delay5/1 -> [VTQD_EnterP_flg]
  [VTQD_ExitP_flg] -> Logical Operator2/4
  [VTQD_EnterP_flg] -> Logical Operator4/4
  [VTQD_ExitP_flg] -> Logical Operator8/4
  [VTQD_ExitP_flg] -> Logical Operator13/4
  [VTQD_GearShiftCMD_enum] -> Equal20/1
  Constant11/1 -> Equal20/2
  Equal20/1 -> Logical Operator19/1
